simulink subsystem "discreteRLC"  (R2023b)
settings: Solver=VariableStepAuto  StartTime=0.0  StopTime=10.0  RelTol=1e-3
values from neighbouring files (symbols this model uses):
  C = 0.5    [code.m]    (also in e03.m)
  L = 2    [code.m]    (also in e03.m)
undefined symbols (not defined in the file or in its folder): DiscIntNeverNeededParam
settings Model: Creator=Anirvan Krishna  LastModifiedBy=Anirvan Krishna

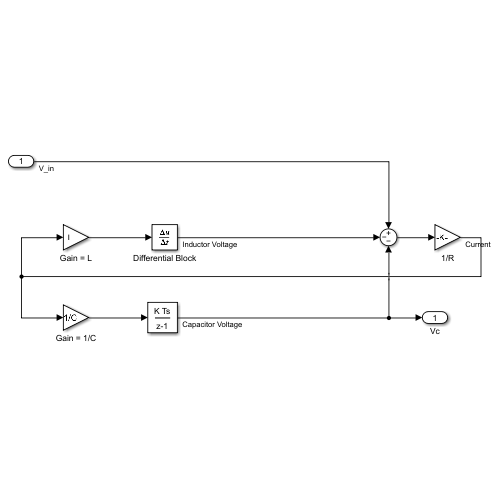
[thumbnail: Simulink's stored preview of the top-level diagram]
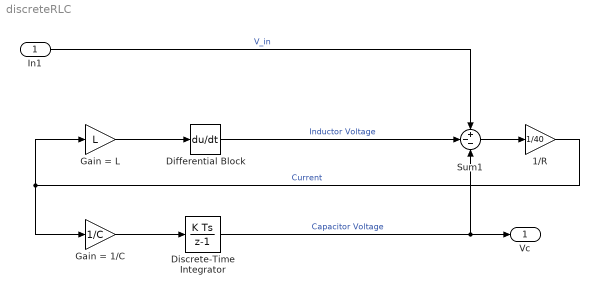
== system discreteRLC ==
  In1 : Inport
  1/R : Gain  Gain=1/40
  Differential Block : Derivative
  Discrete-Time Integrator : DiscreteIntegrator  SampleTime=-1  ICPrevOutput=DiscIntNeverNeededParam  ICPrevScaledInput=DiscIntNeverNeededParam
  Gain = 1/C : Gain  Gain=1/C
  Gain = L : Gain  Gain=L
  Sum1 : Sum  Inputs=+--
  Vc : Outport
  wires:
  Gain = 1/C/1 -> Discrete-Time Integrator/1
  Discrete-Time Integrator/1 -> Vc/1, Sum1/3  "Capacitor Voltage"
  Sum1/1 -> 1/R/1
  1/R/1 -> Gain = 1/C/1, Gain = L/1  "Current"
  In1/1 -> Sum1/1  "V_in"
  Gain = L/1 -> Differential Block/1
  Differential Block/1 -> Sum1/2  "Inductor Voltage"
